simulink model "FuzzyPI_Scenario1_tuned_a_valueTesting"  (R2023a)
settings: Solver=VariableStepAuto  StartTime=0.0  StopTime=16  RelTol=1e-3
model workspace (MAT data in the model file):
  a = Simulink.Parameter
  a.Value = [0.05 0.1 0.5 1]
  a.DataType = 'auto'
  a.Complexity = 'real'
  a.Dimensions = [1 4]
libraries: fuzblock x4, slpidlib x1
settings Model: Creator=minakosm  LastModifiedBy=paris
settings OptimizationCC: ReuseModelBlockBuffer=off

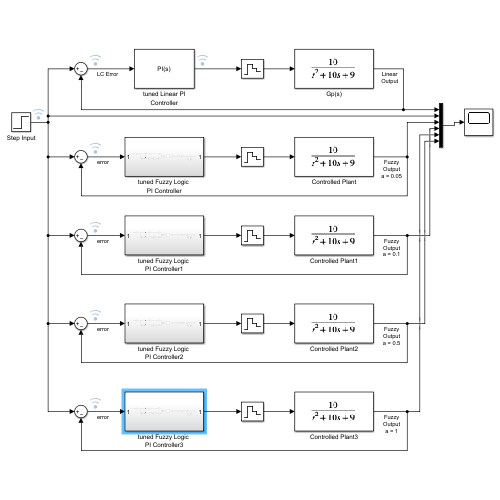
[thumbnail: Simulink's stored preview of the top-level diagram]
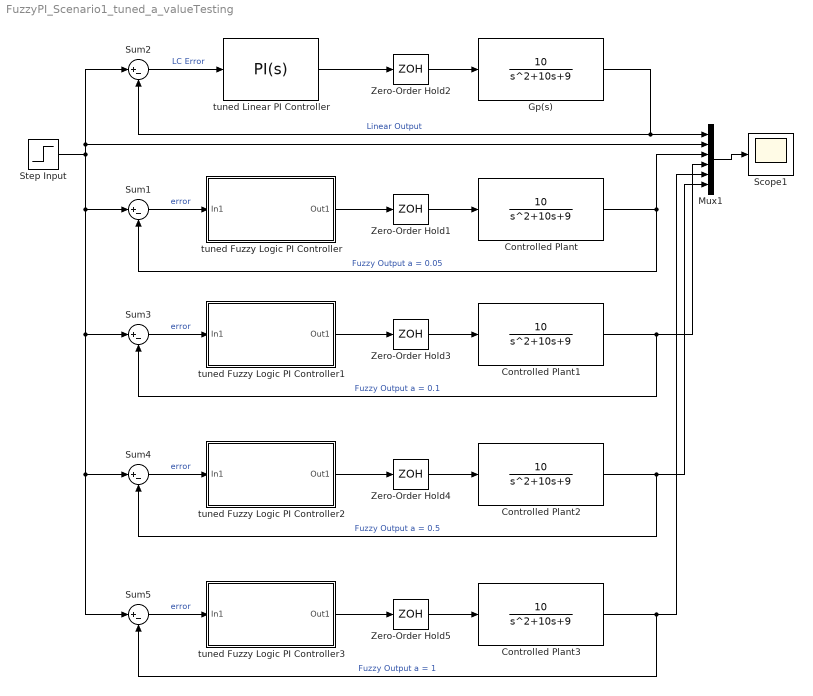
== system FuzzyPI_Scenario1_tuned_a_valueTesting ==
  Controlled Plant{,1..3} (4 alike) : TransferFcn  Numerator=[10]  Denominator=[1 10 9]
  Gp(s) : TransferFcn  Numerator=[10]  Denominator=[1 10 9]
  Mux1 : Mux  Inputs=6
  Scope1 : Scope
  Step Input : Step  Before=50  After=50  SampleTime=0
  Sum{1..5} (5 alike) : Sum  Inputs=|+-
  Zero-Order Hold{1..5} (5 alike) : ZeroOrderHold  SampleTime=-1
  tuned Fuzzy Logic PI Controller : Subsystem
  tuned Fuzzy Logic PI Controller1 : Subsystem
  tuned Fuzzy Logic PI Controller2 : Subsystem
  tuned Fuzzy Logic PI Controller3 : Subsystem
  tuned Linear PI Controller : slpidlib/PID Controller  Controller=PI  Form=Parallel  TimeDomain=Continuous-time  UseExternalTs=off  SampleTime=-1  IntegratorMethod=Forward Euler  FilterMethod=Forward Euler  ControllerParametersSource=internal  P=2.254  I=3  UseKiTs=off  D=0  N=100  UseFilter=on  TunerSelectOption=Transfer Function Based (PID Tuner App)  InitialConditionSource=internal  InitialConditionForIntegrator=0  InitialConditionForFilter=0  DifferentiatorICPrevScaledInput=0  ExternalReset=none  TrackingMode=off  Kt=1  LimitOutput=off  SatLimitsSource=internal  UpperSaturationLimit=inf  LowerSaturationLimit=-inf  LinearizeAsGain=on  AntiWindupMode=none  Kb=1  LimitIntegrator=off  UpperIntegratorSaturationLimit=inf  LowerIntegratorSaturationLimit=-inf  POutMin=[]  POutMax=[]  IOutMin=[]  IOutMax=[]  DOutMin=[]  DOutMax=[]  NOutMin=[]  NOutMax=[]  SumOutMin=[]  SumOutMax=[]  SaturationOutMin=[]  SaturationOutMax=[]  PParamMin=[]  PParamMax=[]  IParamMin=[]  IParamMax=[]  DParamMin=[]  DParamMax=[]  NParamMin=[]  NParamMax=[]  KbParamMin=[]  KbParamMax=[]  KtParamMin=[]  KtParamMax=[]  KbOutMin=[]  KbOutMax=[]  KtOutMin=[]  KtOutMax=[]  IntegratorOutMin=[]  IntegratorOutMax=[]  FilterOutMin=[]  FilterOutMax=[]  SumI1OutMin=[]  SumI1OutMax=[]  SumI2OutMin=[]  SumI2OutMax=[]  SumI3OutMin=[]  SumI3OutMax=[]  SumI4OutMin=[]  SumI4OutMax=[]  SumDOutMin=[]  SumDOutMax=[]  DifferentiatorOutMin=[]  DifferentiatorOutMax=[]  FilterDiffOutCoefMin=[]  FilterDiffOutCoefMax=[]  ReciprocalOutMin=[]  ReciprocalOutMax=[]  SumDenOutMin=[]  SumDenOutMax=[]  SumNumOutMin=[]  SumNumOutMax=[]  DivideOutMin=[]  DivideOutMax=[]  UdiffTsProdOutMin=[]  UdiffTsProdOutMax=[]  NTsProdOutMin=[]  NTsProdOutMax=[]  UintegralTsProdOutMin=[]  UintegralTsProdOutMax=[]  UngainTsProdOutMin=[]  UngainTsProdOutMax=[]  ClampingZeroOutDataTypeStr=Inherit: Inherit via back propagation  ClampingZeroOutMin=[]  ClampingZeroOutMax=[]  FilterDenConstantOutDataTypeStr=Inherit: Inherit via back propagation  FilterDenConstantOutMin=[]  FilterDenConstantOutMax=[]  PCopyOutDataTypeStr=Inherit: Inherit via back propagation  PCopyOutMin=[]  PCopyOutMax=[]  NCopyOutDataTypeStr=Inherit: Inherit via back propagation  NCopyOutMin=[]  NCopyOutMax=[]  IntegratorContinuousStateAttributes=''  IntegratorStateMustResolveToSignalObject=off  IntegratorRTWStateStorageClass=Auto  FilterContinuousStateAttributes=''  FilterStateMustResolveToSignalObject=off  FilterRTWStateStorageClass=Auto  ParallelPVariant=InternalParameters  IdealPVariant=Disabled  IVariant=InternalParameters  DVariant=Disabled  IntegratorVariant=Continuous  SatVariant=Disabled  AWVariant=Passthrough  PCopyVariant=Disabled  TRVariant=Disabled  FdbkBlocksVariant=Forward  IdealPFdbkVariant=Disabled  SatFdbkVariant=Disabled  DerivativeFilterVariant=Disabled  NVariant=Disabled  NCopyVariant=Disabled_SignalSpec  FilterICVariant=Disabled  IntegratorICVariant=InternalICs  ExternalResetVariant=Disabled  TRSumVariant=Passthrough  SumFdbkVariant=Disabled  SumVariant=Sum_PI  TsampFilterVariant=InternalTs  TsampNgainVariant=Passthrough  TsampIntegralVariant=Disabled_SignalSpec  ExternalSaturationOutDataTypeStr=Inherit: Same as second input
  wires:
  Sum1/1 -> tuned Fuzzy Logic PI Controller/1(In1)  "error"
  tuned Fuzzy Logic PI Controller/1(Out1) -> Zero-Order Hold1/1
  Zero-Order Hold1/1 -> Controlled Plant/1
  Controlled Plant/1 -> Sum1/2, Mux1/3  "Fuzzy Output a = 0.05"
  Mux1/1 -> Scope1/1
  Gp(s)/1 -> Sum2/2, Mux1/1  "Linear Output"
  Sum2/1 -> tuned Linear PI Controller/1  "LC Error"
  tuned Linear PI Controller/1 -> Zero-Order Hold2/1
  Zero-Order Hold2/1 -> Gp(s)/1
  Controlled Plant1/1 -> Mux1/4, Sum3/2  "Fuzzy Output a = 0.1"
  tuned Fuzzy Logic PI Controller1/1(Out1) -> Zero-Order Hold3/1
  Sum3/1 -> tuned Fuzzy Logic PI Controller1/1(In1)  "error"
  Zero-Order Hold3/1 -> Controlled Plant1/1
  Controlled Plant2/1 -> Mux1/6, Sum4/2  "Fuzzy Output a = 0.5"
  tuned Fuzzy Logic PI Controller2/1(Out1) -> Zero-Order Hold4/1
  Sum4/1 -> tuned Fuzzy Logic PI Controller2/1(In1)  "error"
  Zero-Order Hold4/1 -> Controlled Plant2/1
  Controlled Plant3/1 -> Mux1/5, Sum5/2  "Fuzzy Output a = 1"
  Step Input/1 -> Sum2/1, Mux1/2, Sum5/1, Sum4/1, Sum3/1, Sum1/1
  tuned Fuzzy Logic PI Controller3/1(Out1) -> Zero-Order Hold5/1
  Sum5/1 -> tuned Fuzzy Logic PI Controller3/1(In1)  "error"
  Zero-Order Hold5/1 -> Controlled Plant3/1

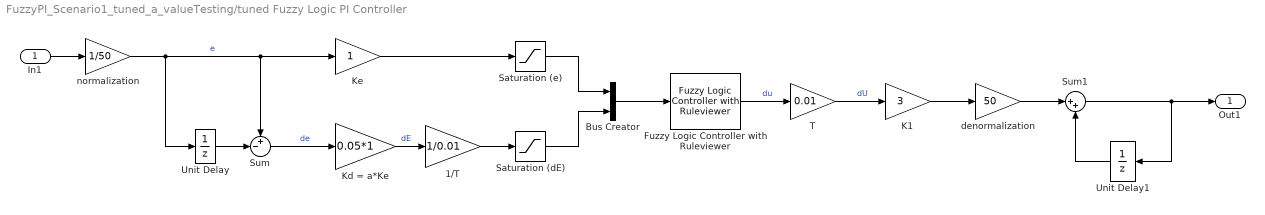
== system FuzzyPI_Scenario1_tuned_a_valueTesting/tuned Fuzzy Logic PI Controller ==
  In1 : Inport
  1/T : Gain  Gain=1/0.01
  Bus Creator : BusCreator  Inputs=2
  Fuzzy Logic Controller with Ruleviewer : fuzblock/Fuzzy Logic  Controller  with Ruleviewer  fismatrix=FuzzyController  Ts=0.01
  K1 : Gain  Gain=3
  Kd = a*Ke : Gain  Gain=0.05*1
  Ke : Gain
  Saturation (dE) : Saturate  UpperLimit=1  LowerLimit=-1
  Saturation (e) : Saturate  UpperLimit=1  LowerLimit=-1
  Sum : Sum  Inputs=+-|
  Sum1 : Sum  Inputs=|++
  T : Gain  Gain=0.01
  Unit Delay : UnitDelay  SampleTime=-1  HasFrameUpgradeWarning=on
  Unit Delay1 : UnitDelay  SampleTime=-1  HasFrameUpgradeWarning=on
  denormalization : Gain  Gain=50
  normalization : Gain  Gain=1/50
  Out1 : Outport
  wires:
  In1/1 -> normalization/1
  K1/1 -> denormalization/1
  Unit Delay/1 -> Sum/2
  Saturation (dE)/1 -> Bus Creator/2
  Sum1/1 -> Out1/1, Unit Delay1/1
  T/1 -> K1/1  "dU"
  Bus Creator/1 -> Fuzzy Logic Controller with Ruleviewer/1
  1/T/1 -> Saturation (dE)/1
  Fuzzy Logic Controller with Ruleviewer/1 -> T/1  "du"
  Saturation (e)/1 -> Bus Creator/1
  Sum/1 -> Kd = a*Ke/1  "de"
  normalization/1 -> Ke/1, Sum/1, Unit Delay/1  "e"
  Ke/1 -> Saturation (e)/1
  Unit Delay1/1 -> Sum1/2
  denormalization/1 -> Sum1/1
  Kd = a*Ke/1 -> 1/T/1  "dE"

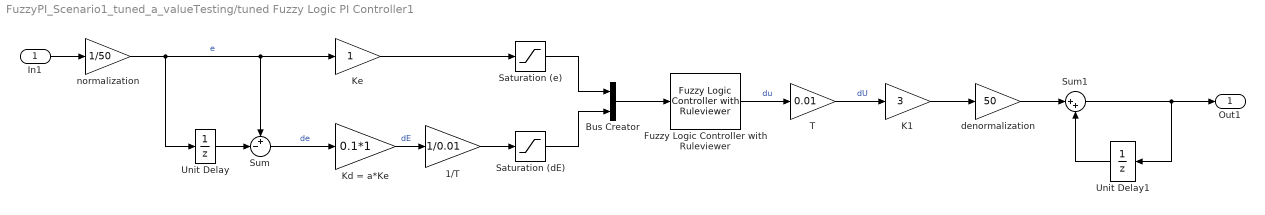
== system FuzzyPI_Scenario1_tuned_a_valueTesting/tuned Fuzzy Logic PI Controller1 ==
  In1 : Inport
  1/T : Gain  Gain=1/0.01
  Bus Creator : BusCreator  Inputs=2
  Fuzzy Logic Controller with Ruleviewer : fuzblock/Fuzzy Logic  Controller  with Ruleviewer  fismatrix=FuzzyController  Ts=0.01
  K1 : Gain  Gain=3
  Kd = a*Ke : Gain  Gain=0.1*1
  Ke : Gain
  Saturation (dE) : Saturate  UpperLimit=1  LowerLimit=-1
  Saturation (e) : Saturate  UpperLimit=1  LowerLimit=-1
  Sum : Sum  Inputs=+-|
  Sum1 : Sum  Inputs=|++
  T : Gain  Gain=0.01
  Unit Delay : UnitDelay  SampleTime=-1  HasFrameUpgradeWarning=on
  Unit Delay1 : UnitDelay  SampleTime=-1  HasFrameUpgradeWarning=on
  denormalization : Gain  Gain=50
  normalization : Gain  Gain=1/50
  Out1 : Outport
  wires:
  In1/1 -> normalization/1
  K1/1 -> denormalization/1
  Unit Delay/1 -> Sum/2
  Saturation (dE)/1 -> Bus Creator/2
  Sum1/1 -> Out1/1, Unit Delay1/1
  T/1 -> K1/1  "dU"
  Bus Creator/1 -> Fuzzy Logic Controller with Ruleviewer/1
  1/T/1 -> Saturation (dE)/1
  Fuzzy Logic Controller with Ruleviewer/1 -> T/1  "du"
  Saturation (e)/1 -> Bus Creator/1
  Sum/1 -> Kd = a*Ke/1  "de"
  normalization/1 -> Ke/1, Sum/1, Unit Delay/1  "e"
  Ke/1 -> Saturation (e)/1
  Unit Delay1/1 -> Sum1/2
  denormalization/1 -> Sum1/1
  Kd = a*Ke/1 -> 1/T/1  "dE"

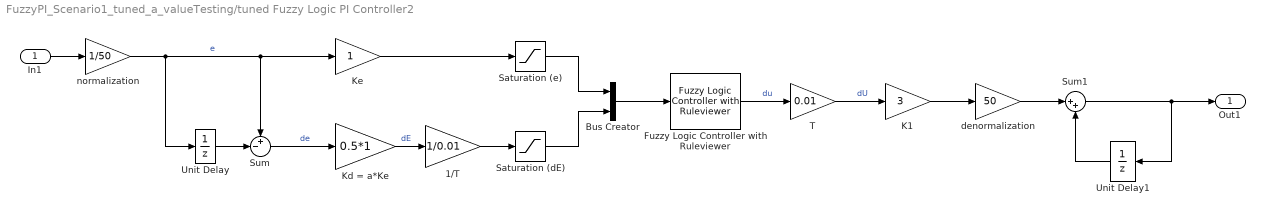
== system FuzzyPI_Scenario1_tuned_a_valueTesting/tuned Fuzzy Logic PI Controller2 ==
  In1 : Inport
  1/T : Gain  Gain=1/0.01
  Bus Creator : BusCreator  Inputs=2
  Fuzzy Logic Controller with Ruleviewer : fuzblock/Fuzzy Logic  Controller  with Ruleviewer  fismatrix=FuzzyController  Ts=0.01
  K1 : Gain  Gain=3
  Kd = a*Ke : Gain  Gain=0.5*1
  Ke : Gain
  Saturation (dE) : Saturate  UpperLimit=1  LowerLimit=-1
  Saturation (e) : Saturate  UpperLimit=1  LowerLimit=-1
  Sum : Sum  Inputs=+-|
  Sum1 : Sum  Inputs=|++
  T : Gain  Gain=0.01
  Unit Delay : UnitDelay  SampleTime=-1  HasFrameUpgradeWarning=on
  Unit Delay1 : UnitDelay  SampleTime=-1  HasFrameUpgradeWarning=on
  denormalization : Gain  Gain=50
  normalization : Gain  Gain=1/50
  Out1 : Outport
  wires:
  In1/1 -> normalization/1
  K1/1 -> denormalization/1
  Unit Delay/1 -> Sum/2
  Saturation (dE)/1 -> Bus Creator/2
  Sum1/1 -> Out1/1, Unit Delay1/1
  T/1 -> K1/1  "dU"
  Bus Creator/1 -> Fuzzy Logic Controller with Ruleviewer/1
  1/T/1 -> Saturation (dE)/1
  Fuzzy Logic Controller with Ruleviewer/1 -> T/1  "du"
  Saturation (e)/1 -> Bus Creator/1
  Sum/1 -> Kd = a*Ke/1  "de"
  normalization/1 -> Ke/1, Sum/1, Unit Delay/1  "e"
  Ke/1 -> Saturation (e)/1
  Unit Delay1/1 -> Sum1/2
  denormalization/1 -> Sum1/1
  Kd = a*Ke/1 -> 1/T/1  "dE"

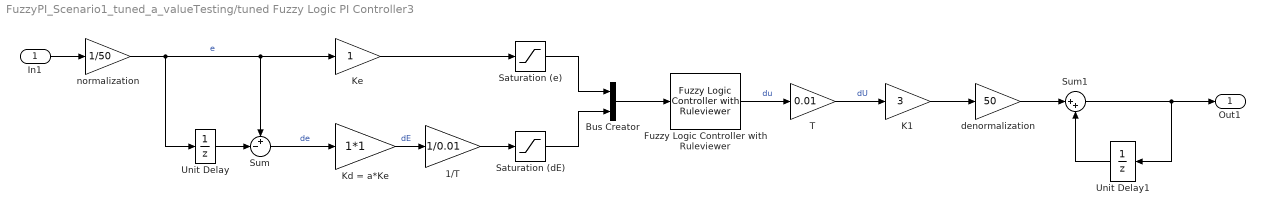
== system FuzzyPI_Scenario1_tuned_a_valueTesting/tuned Fuzzy Logic PI Controller3 ==
  In1 : Inport
  1/T : Gain  Gain=1/0.01
  Bus Creator : BusCreator  Inputs=2
  Fuzzy Logic Controller with Ruleviewer : fuzblock/Fuzzy Logic  Controller  with Ruleviewer  fismatrix=FuzzyController  Ts=0.01
  K1 : Gain  Gain=3
  Kd = a*Ke : Gain  Gain=1*1
  Ke : Gain
  Saturation (dE) : Saturate  UpperLimit=1  LowerLimit=-1
  Saturation (e) : Saturate  UpperLimit=1  LowerLimit=-1
  Sum : Sum  Inputs=+-|
  Sum1 : Sum  Inputs=|++
  T : Gain  Gain=0.01
  Unit Delay : UnitDelay  SampleTime=-1  HasFrameUpgradeWarning=on
  Unit Delay1 : UnitDelay  SampleTime=-1  HasFrameUpgradeWarning=on
  denormalization : Gain  Gain=50
  normalization : Gain  Gain=1/50
  Out1 : Outport
  wires:
  In1/1 -> normalization/1
  K1/1 -> denormalization/1
  Unit Delay/1 -> Sum/2
  Saturation (dE)/1 -> Bus Creator/2
  Sum1/1 -> Out1/1, Unit Delay1/1
  T/1 -> K1/1  "dU"
  Bus Creator/1 -> Fuzzy Logic Controller with Ruleviewer/1
  1/T/1 -> Saturation (dE)/1
  Fuzzy Logic Controller with Ruleviewer/1 -> T/1  "du"
  Saturation (e)/1 -> Bus Creator/1
  Sum/1 -> Kd = a*Ke/1  "de"
  normalization/1 -> Ke/1, Sum/1, Unit Delay/1  "e"
  Ke/1 -> Saturation (e)/1
  Unit Delay1/1 -> Sum1/2
  denormalization/1 -> Sum1/1
  Kd = a*Ke/1 -> 1/T/1  "dE"
